simulink model "PID"  (Simulink 8.5)
settings: Solver=ode3  StartTime=0.0  StopTime=inf  FixedStep=.002  RelTol=1e-3
values from neighbouring files (symbols this model uses):
  arm_home = [ -0.1106   -1.9490   -0.1920    3.1840 ]    [NEW_PID_4DOF.m]    (also in SetPoint_Control.m = [ -0.1106   -1.9490   -0.1920    3.1840    0.2825    0.0969 ; Stochastic_coriolis.m = [  -0.1106   -1.9490   -0.1920    3.1840    0.2825    0.0969; Untitled4.m = [ -0.1106   -1.9490   -0.1920    3.1840    0.2825    0.0969 )
  C = Cjk(q)    [B.m]    (also in DC_motor.m = [1  0  0]; ILC_Grav_Comp.m = [zeros(7,7),eye(7)]; ILC_Grav_Comp_Diff.m = [zeros(7,7),eye(7)]; ILC_Grav_comp_Kalman.m = [zeros(7,7),eye(7)])
  x1 = [[-0.11060;-2;-0.19200;3.1;0.28250;0.09690;-0.27980],zeros(7,n-1)]    [ILC_Grav_Comp.m]    (also in ILC_Grav_Comp_Diff.m; ILC_Grav_comp_Kalman.m; NEW_PID_4DOF.m = alfa*posd(:,1); New_PID.m = alfa*posd(:,1))
undefined symbols (not defined in the file or in its folder): arm_j2mt, arm_m2jp, bit, CAN_init, enc_per_rev, FT_init, MT_init, puck_I_per_Nm, sample_time, Standard, VL1_init, VL2_init, yddel
libraries: slrtlib x11, simulink x8, slrtsoftinglib x7, xpcutilitieslib x4
settings Model: Creator=Matt Courtney  LastModifiedBy=User
settings SolverCC: EnableConcurrentExecution=on
settings OptimizationCC: BlockReduction=off  BooleanDataType=off  OptimizeBlockIOStorage=off  BufferReuse=off  GlobalBufferReuse=off  ExpressionFolding=off  LocalBlockOutputs=off  InitFltsAndDblsToZero=on
settings DebuggingCC: SolverPrmCheckMsg=warning  FcnCallInpInsideContextMsg=UseLocalSettings  StrictBusMsg=Warning
settings HardwareCC: ProdIntDivRoundTo=Zero  ProdEndianess=LittleEndian  ProdLongLongMode=on  ProdHWDeviceType=Generic->32-bit x86 compatible
settings RTWCC: SystemTargetFile=slrt.tlc  TemplateMakefile=slrt_default_tmf  Description=Simulink Real-Time  RTWCompilerOptimization=on
settings SimulinkRealTimeCC: GeneratePreprocessorConditionals=Disable all  xPCisModelTimeout=off  xPCModelTimeoutSecs=10

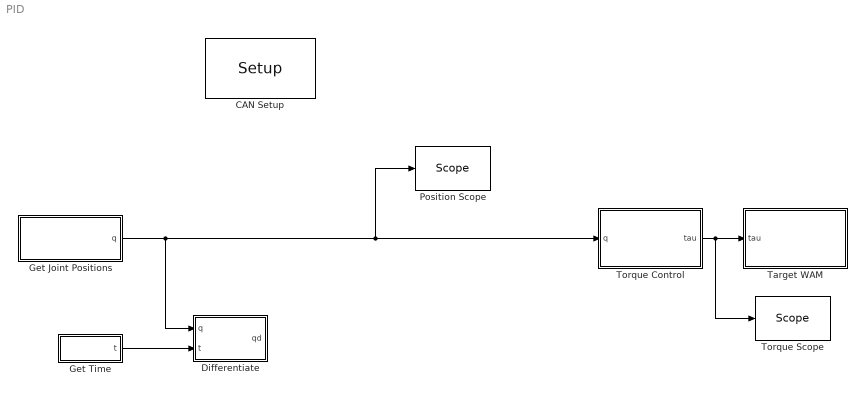
== system PID ==
  "CAN Setup " : slrtsoftinglib/CAN-AC2-PCI SJA 1000/Setup   board=1  can1bus=Highspeed (ISO 11898)  can1Baudrate=1 MBaud  can1UserBR=[1,1,4,3]  can2bus=Highspeed (ISO 11898)  can2Baudrate=1 MBaud  can2UserBR=[1,1,4,3]  init=[VL1_init,VL2_init,CAN_init,FT_init,MT_init]  term=[]  bus_off_out=off  bus_off_rec=Off  ioBaseAddress=-1
  Differentiate : Subsystem
  Get Joint Positions : Subsystem
  Get Time : Subsystem
  Position Scope : slrtlib/Displays and Logging/Scope   scopeno=5  scopetype=Target  autostart=on  viewmode=Numerical  formatstr=['joint_1 %13.8f rad,joint_2 %13.8f rad,joint_3 %13.8f rad,joint_4 %13.8f rad,joint_5 %13.8f rad,joint_6 %13.8f rad,joint_7 %13.8f rad']  grid=on  ylimits=[0,0]  nosamples=1/(10*sample_time)  noprepostsamples=0  interleave=1  triggermode=FreeRun  triggersignal=1  trigsignalfromport=off  triggerlevel=0.0  triggerslope=Either  triggerscope=1  triggersample=0  filename=data.dat  mode=Lazy  writesize=512  autorestart=off  dynamicfilemode=off  maxwritefilesize=512*1024^2
  Target WAM : Subsystem
  Torque Control : Subsystem
  Torque Scope : slrtlib/Displays and Logging/Scope   scopeno=1  scopetype=Target  autostart=on  viewmode=Numerical  formatstr=['joint_1 %10.5f N-m,joint_2 %10.5f N-m,joint_3 %10.5f N-m,joint_4 %10.5f N-m,joint_5 %10.5f N-m,joint_6 %10.5f N-m,joint_7 %10.5f N-m']  grid=on  ylimits=[0,0]  nosamples=1/(10*sample_time)  noprepostsamples=0  interleave=1  triggermode=FreeRun  triggersignal=1  trigsignalfromport=off  triggerlevel=0.0  triggerslope=Either  triggerscope=1  triggersample=0  filename=data.dat  mode=Lazy  writesize=512  autorestart=off  dynamicfilemode=off  maxwritefilesize=512*1024^2
  wires:
  Torque Control/1(tau) -> Target WAM/1(tau), Torque Scope/1
  Get Joint Positions/1(q) -> Differentiate/1(q), Torque Control/1(q), Position Scope/1
  Get Time/1(t) -> Differentiate/2(t)

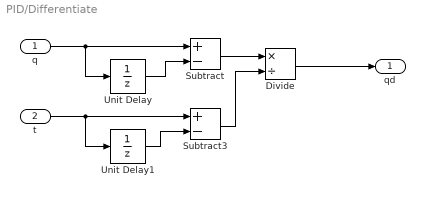
== system PID/Differentiate ==
  q : Inport
  t : Inport  Port=2
  Divide : Product  Inputs=*/
  Subtract : Sum  Inputs=+-
  Subtract3 : Sum  Inputs=+-
  Unit Delay : UnitDelay  SampleTime=-1
  Unit Delay1 : UnitDelay  SampleTime=-1
  qd : Outport
  wires:
  q/1 -> Subtract/1, Unit Delay/1
  t/1 -> Unit Delay1/1, Subtract3/1
  Unit Delay1/1 -> Subtract3/2
  Unit Delay/1 -> Subtract/2
  Subtract/1 -> Divide/1
  Divide/1 -> qd/1
  Subtract3/1 -> Divide/2

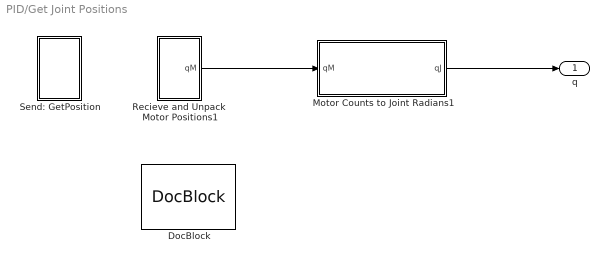
== system PID/Get Joint Positions ==
  DocBlock : simulink/Model-Wide Utilities/DocBlock  DocumentType=Text
  Motor Counts to Joint Radians1 : Subsystem
  Recieve and Unpack  Motor Positions1 : Subsystem
  Send: GetPosition : Subsystem
  q : Outport
  wires:
  Motor Counts to Joint Radians1/1(qJ) -> q/1
  Recieve and Unpack  Motor Positions1/1(qM) -> Motor Counts to Joint Radians1/1(qM)

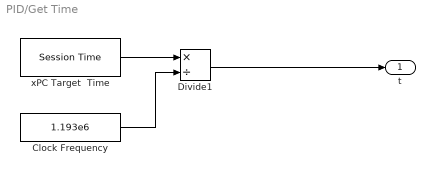
== system PID/Get Time ==
  Clock Frequency : Constant  Value=1.193e6
  Divide1 : Product  Inputs=*/
  "xPC Target  Time " : slrtlib/Target Management/Target Information/Session Time   ts=sample_time
  t : Outport
  wires:
  "xPC Target  Time "/1 -> Divide1/1
  Clock Frequency/1 -> Divide1/2
  Divide1/1 -> t/1

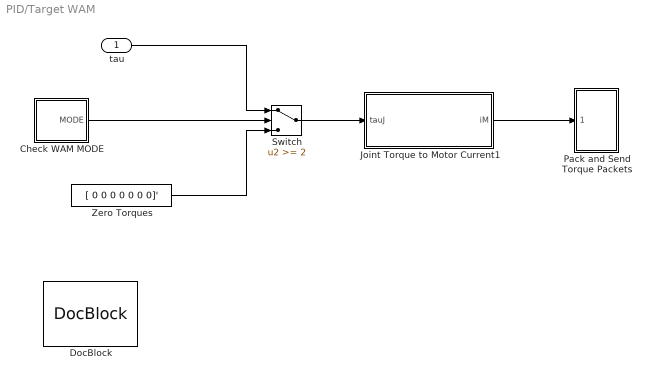
== system PID/Target WAM ==
  tau : Inport
  Check WAM MODE : Subsystem
  DocBlock : simulink/Model-Wide Utilities/DocBlock  DocumentType=Text
      content=|
      | This block does all of the communication with the WAM over the CAN card.
      | First we check the WAM mode to see if it in is Shift-Idle or Shift-Active
      | mode. It is necessary to pass this as output, so that PID knows whether it
      | should be integrating on the error or not. If we are in Shift-Idle mode,
      | we send zero torques. Also in this block, we convert joint torque to motor
      | current using the transformations in the documentation. Then we pack the
      | torque packets into a CAN message and send it.
      |
      | To receive joint positions we also send a CAN message which will respond
      | back with the appropriate information. Once we receive the joint positions,
      | we need to differentiate it to get joint velocities (since the WAM does not
      | have tachometers). Finally, passing it through a moving average of the last
      | n readings removes some of the noise and gives us a smoother velocity
      | signal.
  Joint Torque to Motor Current1 : Subsystem
  Pack and Send Torque Packets : Subsystem
  Switch : Switch  Threshold=2
  Zero Torques : Constant  Value=[ 0 0 0 0 0 0 0]'  OutDataTypeStr=int16
  wires:
  Joint Torque to Motor Current1/1(iM) -> Pack and Send Torque Packets/1(Current)
  Switch/1 -> Joint Torque to Motor Current1/1(tauJ)
  tau/1 -> Switch/1
  Zero Torques/1 -> Switch/3
  Check WAM MODE/1(MODE) -> Switch/2

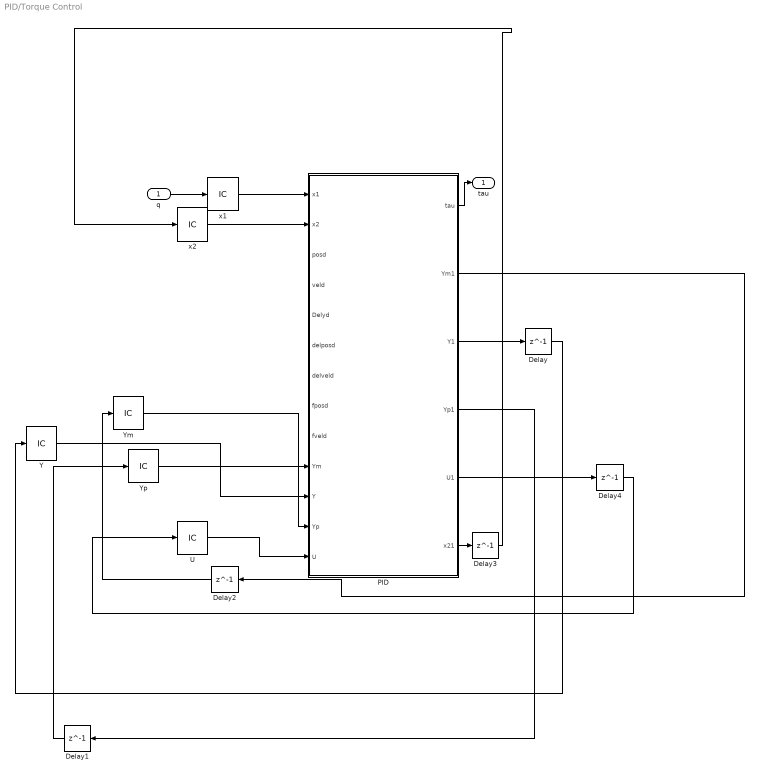
== system PID/Torque Control ==
  q : Inport
  Delay{,1..4} (5 alike) : Delay  DelayLength=1  InitialCondition=0
  PID : MATLAB Function  TreatAsAtomicUnit=on
  U : InitialCondition  Value=[0 0 0 0 0 0 0]
  Y : InitialCondition  Value=[C*[x1' x2']]'
  Ym : InitialCondition  Value=[yddel(:,1)]
  Yp : InitialCondition  Value=[C*[x1' x2']]'
  x1 : InitialCondition  Value=[yddel(:,1)]
  x2 : InitialCondition  Value=[0 0 0 0 0 0 0]
  tau : Outport
  wires:
  PID/1(tau) -> tau/1
  Ym/1 -> PID/10(Ym)
  Y/1 -> PID/11(Y)
  Yp/1 -> PID/12(Yp)
  PID/2(Ym1) -> Delay2/1
  PID/3(Y1) -> Delay/1
  PID/4(Yp1) -> Delay1/1
  Delay/1 -> Y/1
  Delay1/1 -> Yp/1
  Delay2/1 -> Ym/1
  q/1 -> x1/1
  x1/1 -> PID/1(x1)
  PID/6(x21) -> Delay3/1
  Delay3/1 -> x2/1
  PID/5(U1) -> Delay4/1
  Delay4/1 -> U/1
  U/1 -> PID/13(U)
  x2/1 -> PID/2(x2)

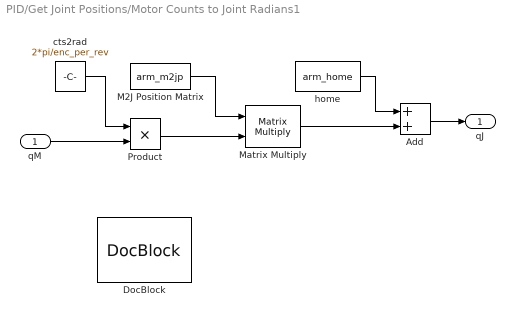
== system PID/Get Joint Positions/Motor Counts to Joint Radians1 ==
  qM : Inport
  Add : Sum
  DocBlock : simulink/Model-Wide Utilities/DocBlock  DocumentType=Text
      content=|
      | Here we do the simple conversion from motor position to joint position,
      | then convert encoder counts to joint radians, then account for the offset
      | in the home position to finally output the joint position in radians. The
      | M2J position matrix can be found in the documentation. Joint 4 has a -18 as
      | opposed to +18 because the motor was reversed at one point during a repair.
      | I believe newer models of the WAM adhere to this -18.
  M2J Position Matrix : Constant  Value=arm_m2jp
  Matrix Multiply : Product  Multiplication=Matrix(*)
  Product : Product  OutMin=[-8192]  OutMax=[8191]  RndMeth=Zero
  cts2rad : Constant  Value=2*pi/enc_per_rev
  home : Constant  Value=arm_home
  qJ : Outport
  wires:
  qM/1 -> Product/2
  Add/1 -> qJ/1
  Matrix Multiply/1 -> Add/2
  home/1 -> Add/1
  cts2rad/1 -> Product/1
  M2J Position Matrix/1 -> Matrix Multiply/1
  Product/1 -> Matrix Multiply/2

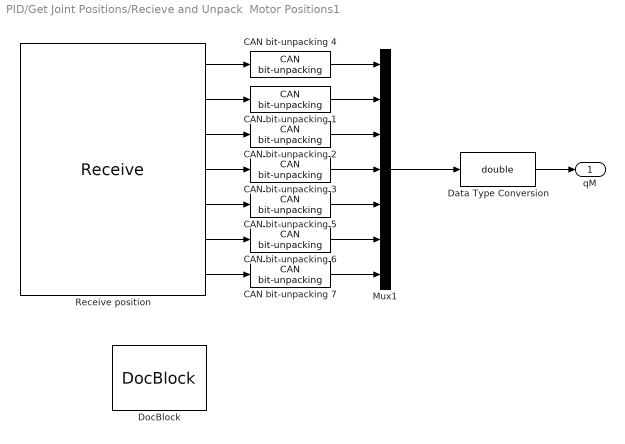
== system PID/Get Joint Positions/Recieve and Unpack  Motor Positions1 ==
  CAN bit-unpacking {1..7} (7 alike) : slrtlib/CAN/Utilities/CAN bit-unpacking   bitpatterns={ [16:23, 8:15, 0:5,-1, -1] }  dtypes={ 'int32'}
  Data Type Conversion : DataTypeConversion  OutDataTypeStr=double
  DocBlock : simulink/Model-Wide Utilities/DocBlock  DocumentType=Text
  Mux1 : Mux  Inputs=7
  "Receive position " : slrtsoftinglib/CAN-AC2-PCI SJA 1000/Receive   board=1  canPort=CAN 1  range=Standard (11-bit)  ids=[bin2dec('10000100011'),bin2dec('10001000011'),bin2dec('10001100011'),bin2dec('10010000011'),bin2dec('10010100011'),bin2dec('10011000011'),bin2dec('10011100011')]  lengths=0  output=Data  inten=on  ts=sample_time  ididx=[0,1,2,3,5,6,7]
  qM : Outport
  wires:
  Mux1/1 -> Data Type Conversion/1
  "Receive position "/1 -> CAN bit-unpacking 4/1
  "Receive position "/2 -> CAN bit-unpacking 1/1
  "Receive position "/3 -> CAN bit-unpacking 2/1
  "Receive position "/4 -> CAN bit-unpacking 3/1
  CAN bit-unpacking 4/1 -> Mux1/1
  CAN bit-unpacking 1/1 -> Mux1/2
  CAN bit-unpacking 2/1 -> Mux1/3
  CAN bit-unpacking 3/1 -> Mux1/4
  Data Type Conversion/1 -> qM/1
  "Receive position "/5 -> CAN bit-unpacking 5/1
  "Receive position "/6 -> CAN bit-unpacking 6/1
  "Receive position "/7 -> CAN bit-unpacking 7/1
  CAN bit-unpacking 5/1 -> Mux1/5
  CAN bit-unpacking 6/1 -> Mux1/6
  CAN bit-unpacking 7/1 -> Mux1/7

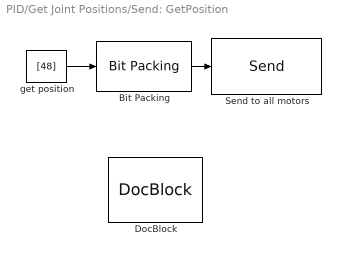
== system PID/Get Joint Positions/Send: GetPosition ==
  Bit Packing : xpcutilitieslib/Bit Packing   MaskBitPatterns={[0:7]}  MaskPackDataType=double  MaskPackDataSize=[1]
  DocBlock : simulink/Model-Wide Utilities/DocBlock  DocumentType=Text
  Send to all motors : slrtsoftinglib/CAN-AC2-PCI SJA 1000/Send   board=1  canPort=CAN 1  range=Standard (11-bit)  ids=1024  sizes=[1]  output=off  ts=sample_time  ididx=[2]
  get position : Constant  Value=[48]  OutDataTypeStr=int8
  wires:
  Bit Packing/1 -> Send to all motors/1
  get position/1 -> Bit Packing/1

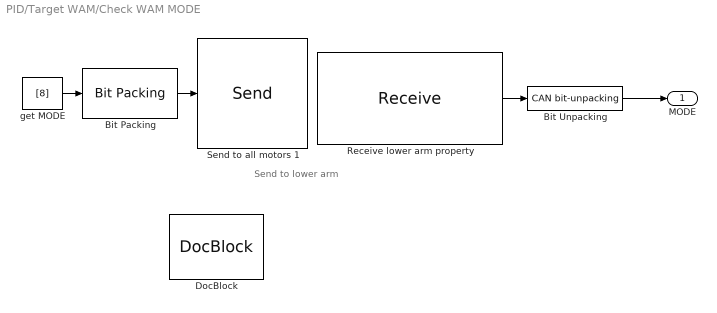
== system PID/Target WAM/Check WAM MODE ==
  note: Send to lower arm
  "Bit Packing " : xpcutilitieslib/Bit Packing   MaskBitPatterns={[0:7]}  MaskPackDataType=double  MaskPackDataSize=[1]
  Bit Unpacking : slrtlib/CAN/Utilities/CAN bit-unpacking   bitpatterns={[16:31]}  dtypes={ 'int16'}
  DocBlock : simulink/Model-Wide Utilities/DocBlock  DocumentType=Text
      content=|
      | Here we send an 8 to the lower arm. Property 8 is the MODE and the
      | 1028 (1 00000 00100) means to "set a lower arm property". Finally we
      | receive the mode property from CAN ID 1158, then do some bit unpacking.
      | All of this is well documentated in the "CAN Communication Spec" of the
      | Barrett documentation.
  Receive lower arm property : slrtsoftinglib/CAN-AC2-PCI SJA 1000/Receive   board=1  canPort=CAN 1  range=Standard (11-bit)  ids=[bin2dec('10010000110')]  lengths=0  output=Data  inten=on  ts=sample_time  ididx=[4]
  Send to all motors 1 : slrtsoftinglib/CAN-AC2-PCI SJA 1000/Send   board=1  canPort=CAN 1  range=Standard (11-bit)  ids=[1028]  sizes=[1]  output=off  ts=sample_time  ididx=[5]
  get MODE : Constant  Value=[8]  OutDataTypeStr=uint8
  MODE : Outport
  wires:
  "Bit Packing "/1 -> Send to all motors 1/1
  Receive lower arm property/1 -> Bit Unpacking/1
  get MODE/1 -> "Bit Packing "/1
  Bit Unpacking/1 -> MODE/1

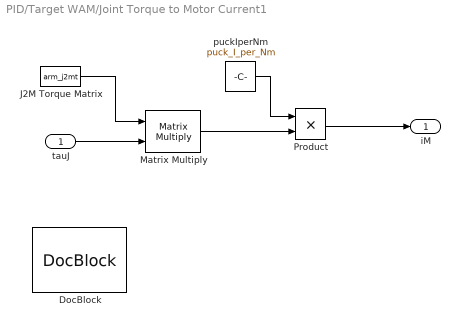
== system PID/Target WAM/Joint Torque to Motor Current1 ==
  tauJ : Inport
  DocBlock : simulink/Model-Wide Utilities/DocBlock  DocumentType=Text
  J2M Torque Matrix : Constant  Value=arm_j2mt
  Matrix Multiply : Product  Multiplication=Matrix(*)
  Product : Product  RndMeth=Zero
  puckIperNm : Constant  Value=puck_I_per_Nm
  iM : Outport
  wires:
  J2M Torque Matrix/1 -> Matrix Multiply/1
  Matrix Multiply/1 -> Product/2
  puckIperNm/1 -> Product/1
  Product/1 -> iM/1
  tauJ/1 -> Matrix Multiply/2

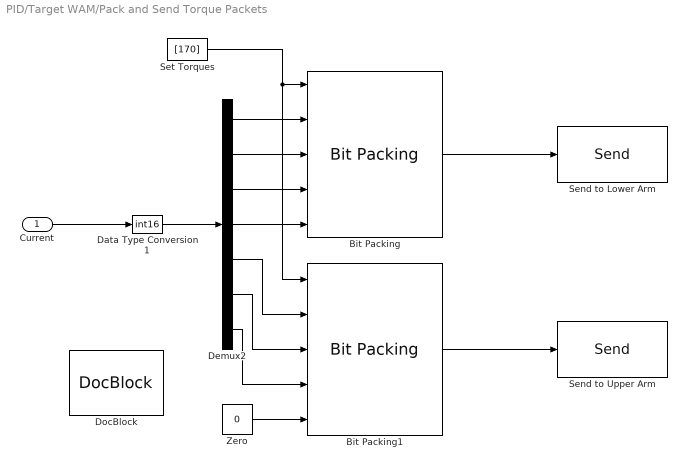
== system PID/Target WAM/Pack and Send Torque Packets ==
  Current : Inport
  Bit Packing : xpcutilitieslib/Bit Packing   MaskBitPatterns={[0:7] [18:23 8:15] [36:39 24:31 16:17] [54:55 40:47 32:35] [56:63 48:53]}  MaskPackDataType=double  MaskPackDataSize=[1]
  Bit Packing1 : xpcutilitieslib/Bit Packing   MaskBitPatterns={[0:7] [18:23 8:15] [36:39 24:31 16:17] [54:55 40:47 32:35] [56:63 48:53]}  MaskPackDataType=double  MaskPackDataSize=[1]
  Data Type Conversion1 : DataTypeConversion  OutMin=[-8191]  OutMax=[8191]  OutDataTypeStr=int16  RndMeth=Zero
  Demux2 : Demux  Outputs=7
  DocBlock : simulink/Model-Wide Utilities/DocBlock  DocumentType=Text
  Send to Lower Arm : slrtsoftinglib/CAN-AC2-PCI SJA 1000/Send   board=1  canPort=CAN 1  range=Standard (11-bit)  ids=bin2dec('10000000001')  sizes=[8]  output=off  ts=sample_time  ididx=[3]
  Send to Upper Arm : slrtsoftinglib/CAN-AC2-PCI SJA 1000/Send   board=1  canPort=CAN 1  range=Standard (11-bit)  ids=bin2dec('10000000010')  sizes=[8]  output=off  ts=sample_time  ididx=[4]
  "Set Torques " : Constant  Value=[170]  OutDataTypeStr=uint8
  Zero : Constant  Value=0  OutDataTypeStr=int16
  wires:
  "Set Torques "/1 -> Bit Packing/1, Bit Packing1/1
  Bit Packing/1 -> Send to Lower Arm/1
  Demux2/1 -> Bit Packing/2
  Demux2/2 -> Bit Packing/3
  Demux2/3 -> Bit Packing/4
  Demux2/4 -> Bit Packing/5
  Current/1 -> Data Type Conversion1/1
  Data Type Conversion1/1 -> Demux2/1
  Bit Packing1/1 -> Send to Upper Arm/1
  Demux2/5 -> Bit Packing1/2
  Demux2/6 -> Bit Packing1/3
  Demux2/7 -> Bit Packing1/4
  Zero/1 -> Bit Packing1/5

== matlab function Torque Control/PID ==
  data: x1 input double; x2 input double; posd input double; tau output double; veld input double; Delyd input double; delposd input double; delveld input double; fposd input double; fveld input double; Ym input double; Y input double; Yp input double; Ym1 output double; Y1 output double; Yp1 output double; U input double; U1 output double; x21 output double
%
% gravComp7DOFNum Compute inverse dynamics via recursive Newton-Euler formulation
%
% Recursive Newton-Euler for standard Denavit-Hartenberg notation.
%

% Copyright (C) 1993-2011, by Peter I. Corke
%
% This file originally was part of The Robotics Toolbox for Matlab (RTB).
%
% http://www.petercorke.com

%
% Simplified from rne_dh for 7DOF WAM to compute only torque from gravity by Hans Vorsteveld
% Does not use structures from RTB, only the RNE algorithm
%

function [tau,Ym1,Y1,Yp1,U1,x21] = PID(x1,x2,posd,veld,Delyd,delposd,delveld,fposd,fveld,Ym,Y,Yp,U)

%-------------------------------------------------------------------------------------
%   SETUP THE ARM
%-------------------------------------------------------------------------------------    
    n = 14;p = 7; q = 14;
    
 Ts=0.002; 




yd = [posd;veld];


 

%initial conditions
%x1 = [-0.11060;-1.949;-0.1920;3.1840;0.2825;0.09690;-0.27980];
%x2 = zeros(7,1);
%U = zeros(7,1);
Ae = (1-Ts)*eye(n);
C= eye(14);
Ce = C;
Iq = eye(q);
Oq = zeros(q);
H = [Iq Oq Oq -Ce*Ae;Iq Oq Oq zeros(q,n);Oq Iq Oq zeros(q,n);zeros(n,q) zeros(n,q) zeros(n,q) Ae];
Ib = zeros(3*q,3*q+n);
for k11 = 1:3*q,Ib(k11,k11) = 1;end
sig = 1e-4;
sigR = sig;
sigQ = 1e-3;
P = 1e-8*eye(3*q+n);
Rb = (sigR^2)*diag(1*ones(3*q,1));
Q = sigQ^2*eye(n);
%X = [x1' x2']';
%Y = C*X;
%Yp = Y;




 Be = Ts*[zeros(7,7);inv(D(x1))];
    Delyd
    Del2yd = Delyd*Delyd';
   
    Gd = [Del2yd Oq Oq zeros(q,n); Oq Oq Oq zeros(q,n); Oq Oq Oq zeros(q,n);zeros(n,q) zeros(n,q) zeros(n,q) Q];
   
    
    
    EE = [Ce*Be;zeros(q,p);zeros(q,p);-Be];
    K = inv(EE'*EE)*EE'*H*P*Ib'*inv(Ib*P*Ib' + Rb);
    PHI = H - EE*K*Ib;

     P = PHI*P*PHI' + EE*K*Rb*K'*EE' + Gd;
    K1 = K(:,1:q);
    K2 = K(:,q+1:2*q);
    K3 = K(:,2*q+1:3*q);
    
    
      %  E = yd - Y ;
       % Ep = ydfut-Yp ;
        %U = U + K1*Ep + K2*E;
        %Ym = Y;
        %Y = Yp;
         %x_1 = x1 ;
       
         %x_11 = x_1; %Since at t=0, velocity is zero
        %XX2 = zeros(7,1);
        %x_22= (-inv(D(x_1))*(transpose(G(x_1)))+ inv(D(x_1))*U)*Ts + XX2 ;
        %Yp = [x_11' x_22']';
       
    
        Em = yddel - Ym ;
        E = yd - Y ;
        Ep = ydfut-Yp ;
        U = U + K1*Ep + K2*E + K3*Em;
        Ym = Y;
        Y = Yp;
        
        x_1 = x1
        
         %
        pos_meas = q ; % In experimental work you do not add noise instead you only use measurement of position
        x_11 =  x_2*Ts + pos_meas; % Here we are estimating position using the extimate of x2 and measurement of x1 at present time
        
        XX2 = (x_11-x_1)/Ts; %
        x_22= (-inv(D(pos_meas))*(transpose(G(pos_meas)))+ inv(D(pos_meas))*U)*Ts + XX2 ;
       
       
        
        Yp = [x_11' x_22']';
    
   
end 

function T = getTransformDH(a,d,alpha,q)
    ct = cos(q);
    st = sin(q);
    cb = cos(alpha);
    sb = sin(alpha);
    
    T = [ ct, -st*cb,  st*sb, a*ct;
          st,  ct*cb, -ct*sb, a*st;
          0, sb, cb, d;
          0, 0, 0, 1 ];
end
